simulink model "only_position"  (R2019a)
settings: Solver=FixedStepAuto  StartTime=0.0  StopTime=20  FixedStep=0.01  RelTol=1e-3
settings Model: Creator=Duong  LastModifiedBy=Duong

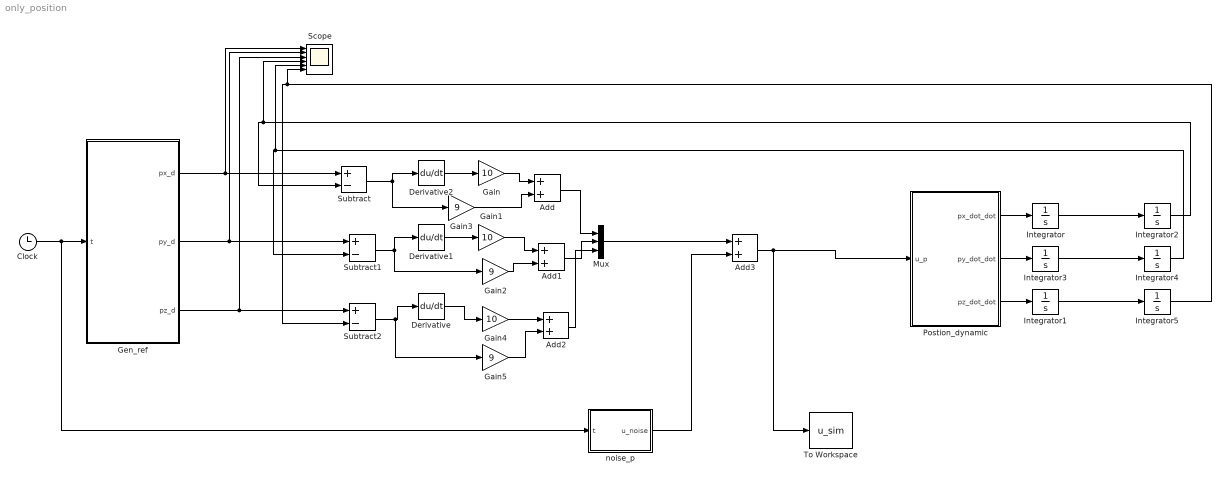
== system only_position ==
  Add{,1..3} (4 alike) : Sum
  Clock : Clock
  Derivative : Derivative
  Derivative1 : Derivative
  Derivative2 : Derivative
  Gain : Gain  Gain=10
  Gain1 : Gain  Gain=10
  Gain2 : Gain  Gain=9
  Gain3 : Gain  Gain=9
  Gain4 : Gain  Gain=10
  Gain5 : Gain  Gain=9
  "Gen_ref " : MATLAB Function  TreatAsAtomicUnit=on
  Integrator{,1..5} (6 alike) : Integrator
  Mux : Mux  Inputs=3
  "Postion_dynamic " : MATLAB Function  TreatAsAtomicUnit=on
  Scope : Scope  NumInputPorts=6
  Subtract : Sum  Inputs=+-
  Subtract1 : Sum  Inputs=+-
  Subtract2 : Sum  Inputs=+-
  To Workspace : ToWorkspace  VariableName=u_sim  SampleTime=-1
      settings: Save2DSignal=2-D array (concatenate along first dimension)
  "noise_p " : MATLAB Function  TreatAsAtomicUnit=on
  wires:
  Clock/1 -> "noise_p "/1(t), "Gen_ref "/1(t)
  "Postion_dynamic "/1(px_dot_dot) -> Integrator/1
  Integrator/1 -> Integrator2/1
  "Postion_dynamic "/2(py_dot_dot) -> Integrator3/1
  Integrator3/1 -> Integrator4/1
  "Postion_dynamic "/3(pz_dot_dot) -> Integrator1/1
  Integrator1/1 -> Integrator5/1
  "Gen_ref "/1(px_d) -> Scope/1, Subtract/1
  "Gen_ref "/2(py_d) -> Scope/2, Subtract1/1
  "Gen_ref "/3(pz_d) -> Subtract2/1, Scope/3
  Integrator2/1 -> Scope/4, Subtract/2
  Integrator4/1 -> Scope/5, Subtract1/2
  Integrator5/1 -> Scope/6, Subtract2/2
  Subtract/1 -> Derivative2/1, Gain3/1
  Derivative2/1 -> Gain/1
  Gain/1 -> Add/1
  Subtract1/1 -> Gain2/1, Derivative1/1
  Derivative1/1 -> Gain1/1
  Gain1/1 -> Add1/1
  Gain2/1 -> Add1/2
  Subtract2/1 -> Gain5/1, Derivative/1
  Derivative/1 -> Gain4/1
  Gain4/1 -> Add2/1
  Gain5/1 -> Add2/2
  Add/1 -> Mux/1
  Add1/1 -> Mux/2
  Add2/1 -> Mux/3
  Gain3/1 -> Add/2
  Mux/1 -> Add3/1
  "noise_p "/1(u_noise) -> Add3/2
  Add3/1 -> To Workspace/1, "Postion_dynamic "/1(u_p)

== matlab function only_position/Postion_dynamic  ==
  data: u_p input; px_dot_dot output; py_dot_dot output; pz_dot_dot output
function [px_dot_dot, py_dot_dot, pz_dot_dot] = fcn(u_p)
px=0;
py=0;
pz=0;
p_dot_dot=zeros(3,1);
    % dXp = A_*Xp + B_*u_;
 m = 2; kw = 1; g = 9.8;
 p_dot_dot=kw/m*u_p;
 px_dot_dot=p_dot_dot(1);
 py_dot_dot=p_dot_dot(2);
 pz_dot_dot=p_dot_dot(3);
 
    
end

function a = e(m, n)
    % Create a (m x 1) vector with 1 in the n th element, and 0s elsewhere
    % m >= n
    a = zeros(m, 1);
    a(n) = 1;
end

== matlab function only_position/Gen_ref  ==
  data: t input; px_d output; py_d output; pz_d output
function [px_d, py_d, pz_d] = fcn(t)
% xp_d = [2*sin(a*t) 2*a*cos(a*t) 2*cos(a*t) -2*a*sin(a*t) 0.8*t 0.8];
a=0.5;
px_d=2*sin(a*t);
py_d=2*cos(a*t);
pz_d=0.8*t;

== matlab function only_position/noise_p  ==
  data: t input; u_noise output
function u_noise = fcn(t)
u_noise=zeros(3,1);
noise=load('noise_gud1.mat');
noise_freq=noise.noise_freq;
freqNum = size(noise_freq,2);
for idx=1:freqNum
    u_noise = u_noise + sin(noise_freq(:,idx)*t);
end
